simulink model "imuTester"  (R2024b)
settings: Solver=FixedStepAuto  StartTime=0.0  StopTime=8000  FixedStep=1/imuHz  RelTol=1e-3
InitFcn:
  | accelParamFile = './Resources/Calibrations/accel_accel0_20251211_allan_stable.mat';
  | gyroParamFile = './Resources/Calibrations/gyro_gyro0_20251211_allan.mat';
  | 
  | accelCalib = load(accelParamFile);
  | gyroCalib = load(gyroParamFile);
  | 
  | imuHz = 8000;
undefined symbols (not defined in the file): fractalcoef
libraries: mspsensorlib x1
settings Model: Creator=Alyssa  LastModifiedBy=Alyssa

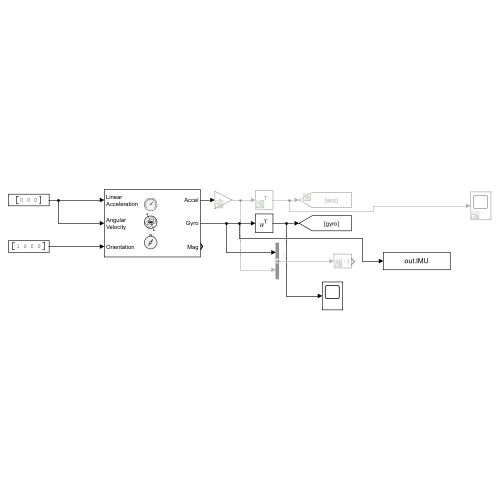
[thumbnail: Simulink's stored preview of the top-level diagram]
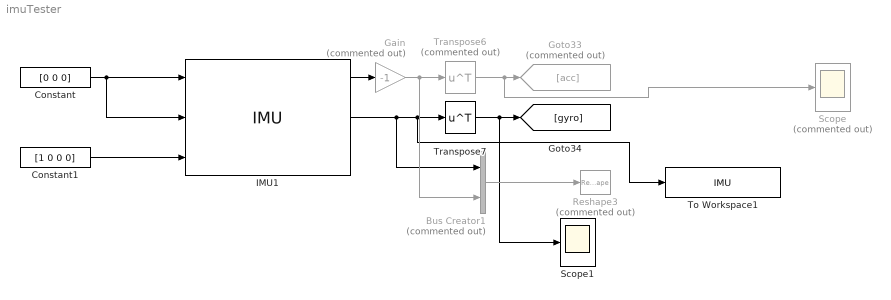
== system imuTester ==
  Bus Creator1 : BusCreator  Commented=on  Inputs=2
  Constant : Constant  Value=[0 0 0]  VectorParams1D=off
  Constant1 : Constant  Value=[1 0 0 0]  VectorParams1D=off
  Gain : Gain  Commented=on  Gain=-1
  Goto33 : Goto  Commented=on  GotoTag=acc
  IMU1 : mspsensorlib/IMU  DispRefFrame=NED  TemperaturePort=off  Temperature=25  MagneticFieldPort=off  MagneticFieldNED=[25.015, -4.798, -22.615];%[ 27.5550, -2.4169, -16.0849 ]  MagneticFieldENU=[ -2.4169, 27.5550, 16.0849 ]  SeedDouble=67  SimulateUsing=Interpreted execution  AccelParamsMeasurementRange=accelCalib.max  AccelParamsResolution=accelCalib.res  AccelParamsConstantBias=accelCalib.simBias  AccelParamsAxesMisalignment=accelCalib.skew  AccelParamsNoiseDensity=accelCalib.vrw  AccelParamsBiasInstability=accelCalib.bi  AccelParamsBiasInstabilityNumerator=fractalcoef().Numerator  AccelParamsBiasInstabilityDenominator=fractalcoef().Denominator  AccelParamsRandomWalk=accelCalib.rrw  AccelParamsNoiseType=double-sided  AccelParamsTemperatureBias=[ 0, 0, 0 ]  AccelParamsTemperatureScaleFactor=[ 0, 0, 0 ]  GyroParamsMeasurementRange=gyroCalib.max  GyroParamsResolution=gyroCalib.res  GyroParamsConstantBias=gyroCalib.simBias  GyroParamsAxesMisalignment=gyroCalib.skew  GyroParamsAccelerationBias=[ 0, 0, 0 ]  GyroParamsNoiseDensity=gyroCalib.arw  GyroParamsBiasInstability=gyroCalib.bi  GyroParamsBiasInstabilityNumerator=fractalcoef().Numerator  GyroParamsBiasInstabilityDenominator=fractalcoef().Denominator  GyroParamsRandomWalk=gyroCalib.rrw  GyroParamsNoiseType=double-sided  GyroParamsTemperatureBias=[ 0, 0, 0 ]  GyroParamsTemperatureScaleFactor=[ 0, 0, 0 ]  MagParamsMeasurementRange=Inf  MagParamsResolution=0  MagParamsConstantBias=[ 0, 0, 0 ]  MagParamsAxesMisalignment=[ 100, 0, 0; 0, 100, 0; 0, 0, 100 ]  MagParamsNoiseDensity=[ 0, 0, 0 ]  MagParamsBiasInstability=[ 0, 0, 0 ]  MagParamsBiasInstabilityNumerator=fractalcoef().Numerator  MagParamsBiasInstabilityDenominator=fractalcoef().Denominator  MagParamsRandomWalk=[ 0, 0, 0 ]  MagParamsNoiseType=double-sided  MagParamsTemperatureBias=[ 0, 0, 0 ]  MagParamsTemperatureScaleFactor=[ 0, 0, 0 ]
  Reshape3 : Reshape  Commented=on
  Scope : Scope  Commented=on
  Scope1 : Scope
  To Workspace1 : ToWorkspace  VariableName=IMU  SaveFormat=Structure With Time  SampleTime=1/imuHz
  Transpose6 : Math  Commented=on  Operator=transpose
  Transpose7 : Math  Operator=transpose
  wires:
  IMU1/2 -> To Workspace1/1, Transpose7/1, Bus Creator1/1
  IMU1/1 -> Gain/1
  Constant/1 -> IMU1/1, IMU1/2
  Gain/1 -> Bus Creator1/2, Transpose6/1
  Transpose6/1 -> Scope/1, Goto33/1
  Transpose7/1 -> Scope1/1, [gyro]
  Bus Creator1/1 -> Reshape3/1
  Constant1/1 -> IMU1/3
